simulink subsystem "untitled"  (R2025b)
settings: Solver=VariableStepAuto  StartTime=0.0  StopTime=10.0  RelTol=1e-3
libraries: simulink x1
settings Model: Creator=Sneha Shree K  LastModifiedBy=Sneha Shree K

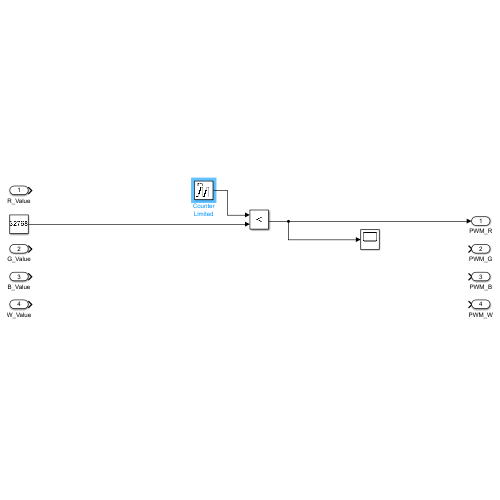
[thumbnail: Simulink's stored preview of the top-level diagram]
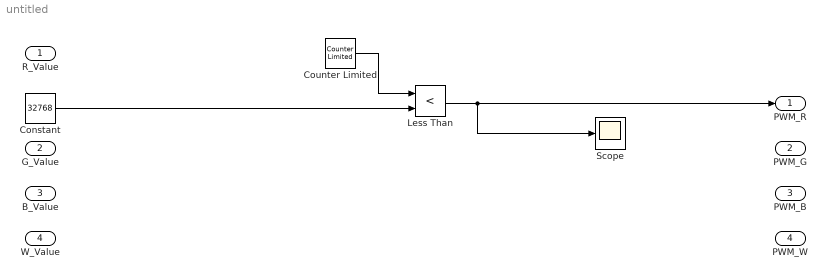
== system untitled ==
  R_Value : Inport
  G_Value : Inport  Port=2
  B_Value : Inport  Port=3
  W_Value : Inport  Port=4
  Constant : Constant  Value=32768  OutDataTypeStr=uint16
  Counter Limited : simulink/Sources/Counter Limited  uplimit=65535  tsamp=1e-6
  Less Than : RelationalOperator  Operator=<  OutDataTypeStr=boolean  RndMeth=Simplest  InputSameDT=off
  Scope : Scope
  PWM_R : Outport
  PWM_G : Outport  Port=2
  PWM_B : Outport  Port=3
  PWM_W : Outport  Port=4
  wires:
  Counter Limited/1 -> Less Than/1
  Less Than/1 -> Scope/1, PWM_R/1
  Constant/1 -> Less Than/2
